simulink model "Simulink_Part_A"  (R2019b)
settings: Solver=VariableStepAuto  StartTime=0.0  StopTime=10.0  RelTol=1e-3
settings Model: Creator=matvey  LastModifiedBy=matvey

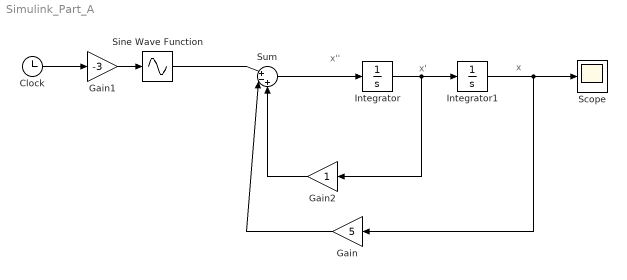
== system Simulink_Part_A ==
  note: x'
  note: x
  note: x''
  Clock : Clock
  Gain : Gain  Gain=5
  Gain1 : Gain  Gain=-3
  Gain2 : Gain
  Integrator : Integrator
  Integrator1 : Integrator  InitialCondition=-5
  Scope : Scope
  Sine Wave Function : Sin  TimeSource=Use external signal  SampleTime=0
  Sum : Sum  Inputs=|+-+
  wires:
  Integrator/1 -> Integrator1/1, Gain2/1
  Sum/1 -> Integrator/1
  Gain/1 -> Sum/2
  Clock/1 -> Gain1/1
  Gain1/1 -> Sine Wave Function/1
  Integrator1/1 -> Scope/1, Gain/1
  Gain2/1 -> Sum/3
  Sine Wave Function/1 -> Sum/1
